simulink model "TestUDP"  (R2015b)
settings: Solver=ode1  SolverMode=SingleTasking  StartTime=0.0  StopTime=inf  FixedStep=0.02  RelTol=1e-3
libraries: xpcutilitieslib x1, xpcrtudplib x1
settings Model: Creator=root  LastModifiedBy=root

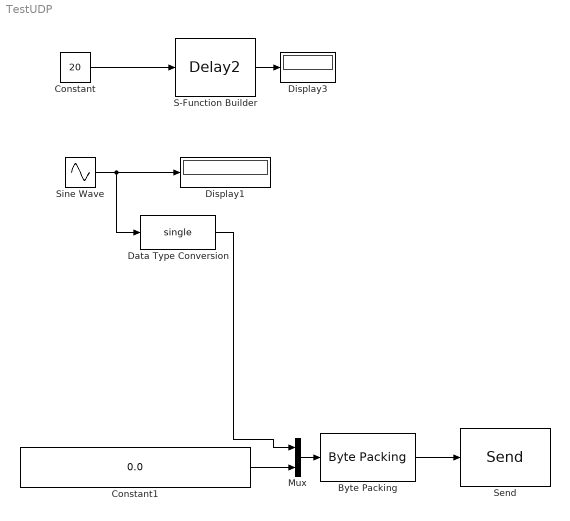
== system TestUDP ==
  "Byte Packing " : xpcutilitieslib/Byte Packing   MaskPackedDataType=uint8  MaskUnpackedDataTypes={'single'}  MaskAlignment=1
  Constant : Constant  Value=20  OutDataTypeStr=uint32  SampleTime=-1
  Constant1 : Constant  Value=0.0  OutDataTypeStr=single  SampleTime=-1
  Data Type Conversion : DataTypeConversion  OutDataTypeStr=single
  Display1 : Display
  Display3 : Display
  Mux : Mux  Inputs=2
  S-Function Builder : S-Function  InitFcn=try, set_param(gcb,'FunctionName','Delay2'), end  FunctionName=Delay2  SFunctionModules=Delay2_wrapper  SFunctionDeploymentMode=off  EnableBusSupport=off  mask(S-Function Builder){}
      mask help: Simulink:masks:SFunctionBuilder_MD
      mask init:
      | val = [[.9  0.75 0.75 1 1 .9 .9 1]',[1 1 0.75 0.75 .9 .9 1 .9]'];try , sys = get_param(gcb,'SfunBuilderFcnName');if isempty(sys), sys = get_param(gcb,'FunctionName'); end,catch, sys = get_param(gcb,'FunctionName'); end
      settings: CopyFcn=set_param(gcbh,'LinkStatus','none')  PreSaveFcn=try, set_param(gcb,'FunctionName','Delay2'), end  OpenFcn=sfunctionwizard(gcbh)
      mask Display: plot(val(:,1),val(:,2)),disp(sys), port_label('input',1,'u0')
  "Send " : xpcrtudplib/Legacy UDP/Send   ipAddress=127.0.0.1  ipPort=12002  localPort=-1  vblLen=off  sampletime=-1
  Sine Wave : Sin  Amplitude=0.5  Bias=0.5
  wires:
  Constant/1 -> S-Function Builder/1
  Sine Wave/1 -> Data Type Conversion/1, Display1/1
  S-Function Builder/1 -> Display3/1
  "Byte Packing "/1 -> "Send "/1
  Mux/1 -> "Byte Packing "/1
  Constant1/1 -> Mux/2
  Data Type Conversion/1 -> Mux/1
